simulink model "Controller_Disc2018"  (R2018b)
settings: Solver=ode8  StartTime=0.0  StopTime=100  FixedStep=1e-4  RelTol=1e-3
undefined symbols (not defined in the file or in its folder): DiscIntNeverNeededParam
libraries: simulink x2
settings Model: Creator=yarat  LastModifiedBy=uidr9910
settings SolverCC: AlgebraicLoopSolver=LineSearch
settings DataIOCC: ReturnWorkspaceOutputs=on

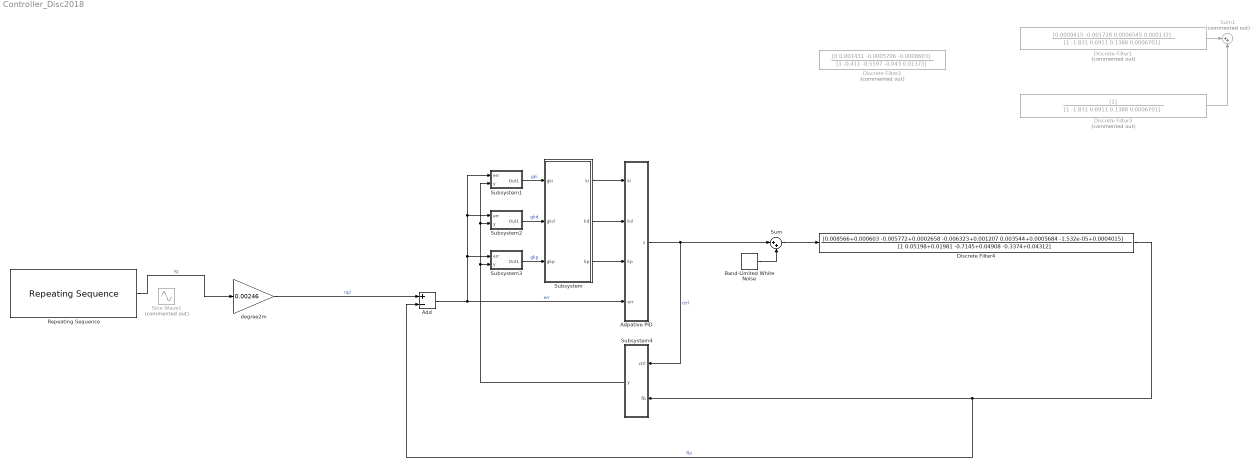
== system Controller_Disc2018 ==
  Add : Sum  Inputs=+-
  Adpative PID : Subsystem
  Band-Limited White Noise : simulink/Sources/Band-Limited White Noise  Cov=[0.00002]  Ts=0.1  seed=[23341]
  Discrete Filter1 : DiscreteFilter  Commented=on  Numerator=[0.0009415 -0.001728 0.0006545 0.000132]  Denominator=[1 -1.831 0.6911 0.1388 0.0006701]  FilterStructure=Direct form I  SampleTime=0.0001
  Discrete Filter2 : DiscreteFilter  Commented=on  Numerator=[0 0.001431 -0.0005706 -0.0008603]  Denominator=[1 -0.411 -0.5597 -0.043 0.01373]  FilterStructure=Direct form I  SampleTime=0.0001
  Discrete Filter3 : DiscreteFilter  Commented=on  Denominator=[1 -1.831 0.6911 0.1388 0.0006701]  FilterStructure=Direct form I  SampleTime=0.0001
  Discrete Filter4 : DiscreteFilter  Numerator=[0.008566+0.000603 -0.005772+0.0002658 -0.006323+0.001207 0.003544+0.0005684 -1.532e-05+0.0004015]  Denominator=[1 0.05198+0.01981 -0.7145+0.04908 -0.3374+0.04312]  FilterStructure=Direct form I  SampleTime=0.0001
  Repeating Sequence : simulink/Sources/Repeating Sequence  rep_seq_t=[0 3 3.01 6 6.01 9 9.01 12]*5  rep_seq_y=[1 1 0 0 -1 -1 0 0]*2
  Sine Wave1 : Sin  Commented=on  Amplitude=2  Frequency=0.5  SampleTime=0
  Subsystem : Subsystem
  Subsystem1 : Subsystem
  Subsystem2 : Subsystem
  Subsystem3 : Subsystem
  Subsystem4 : Subsystem
  Sum : Sum  Inputs=|++
  Sum1 : Sum  Commented=on  Inputs=|++
  degree2m : Gain  Gain=0.00246
  wires:
  degree2m/1 -> Add/1  "rq2"
  Add/1 -> Adpative PID/4(err), Subsystem1/1(err), Subsystem2/1(err), Subsystem3/1(err)  "err"
  Subsystem1/1(Out1) -> Subsystem/1(gki)  "gki"
  Subsystem2/1(Out1) -> Subsystem/2(gkd)  "gkd"
  Subsystem3/1(Out1) -> Subsystem/3(gkp)  "gkp"
  Subsystem/1(ki) -> Adpative PID/1(ki)
  Subsystem/2(kd) -> Adpative PID/2(kd)
  Subsystem/3(kp) -> Adpative PID/3(kp)
  Subsystem4/1(y) -> Subsystem3/2(y), Subsystem2/2(y), Subsystem1/2(y)
  Band-Limited White Noise/1 -> Sum/2
  Adpative PID/1(ctrl) -> Sum/1, Subsystem4/1(ctrl)  "ctrl"
  Sum/1 -> Discrete Filter4/1
  Discrete Filter4/1 -> Add/2, Subsystem4/2(fb)  "fbi"
  Repeating Sequence/1 -> degree2m/1  "rq"
  Discrete Filter1/1 -> Sum1/1
  Discrete Filter3/1 -> Sum1/2

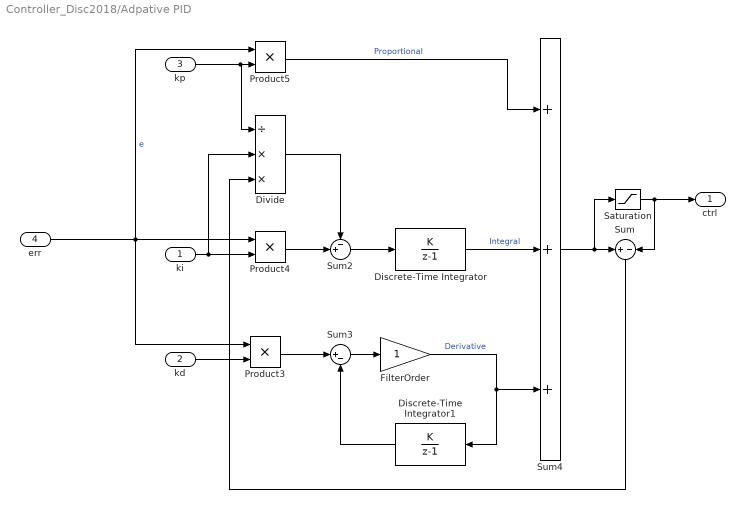
== system Controller_Disc2018/Adpative PID ==
  ki : Inport
  kd : Inport  Port=2
  kp : Inport  Port=3
  err : Inport  Port=4
  Discrete-Time Integrator : DiscreteIntegrator  IntegratorMethod=Accumulation: Forward Euler  gainval=0.001  SampleTime=-1  ICPrevOutput=DiscIntNeverNeededParam  ICPrevScaledInput=DiscIntNeverNeededParam
  Discrete-Time Integrator1 : DiscreteIntegrator  IntegratorMethod=Accumulation: Forward Euler  gainval=0.001  SampleTime=-1  ICPrevOutput=DiscIntNeverNeededParam  ICPrevScaledInput=DiscIntNeverNeededParam
  Divide : Product  Inputs=/**
  FilterOrder : Gain  SaturateOnIntegerOverflow=on  OutDataTypeStr=Inherit: Same as input  ParamDataTypeStr=Inherit: Same as input
  Product3 : Product
  Product4 : Product
  Product5 : Product
  Saturation : Saturate  UpperLimit=100  LowerLimit=-100
  Sum : Sum  Inputs=+|-
  Sum2 : Sum  Inputs=-+|
  Sum3 : Sum  Inputs=|+-
  Sum4 : Sum  Inputs=+++  InputSameDT=on  SaturateOnIntegerOverflow=on  OutDataTypeStr=Inherit: Same as first input
  ctrl : Outport
  wires:
  Discrete-Time Integrator/1 -> Sum4/2  "Integral"
  Discrete-Time Integrator1/1 -> Sum3/2
  Sum/1 -> Divide/3
  Sum2/1 -> Discrete-Time Integrator/1
  Product3/1 -> Sum3/1
  Sum3/1 -> FilterOrder/1
  Product4/1 -> Sum2/2
  FilterOrder/1 -> Sum4/3, Discrete-Time Integrator1/1  "Derivative"
  Product5/1 -> Sum4/1  "Proportional"
  Saturation/1 -> ctrl/1, Sum/2
  err/1 -> Product4/1, Product3/1, Product5/1  "e"
  Sum4/1 -> Saturation/1, Sum/1
  kp/1 -> Divide/1, Product5/2
  ki/1 -> Product4/2, Divide/2
  kd/1 -> Product3/2
  Divide/1 -> Sum2/1

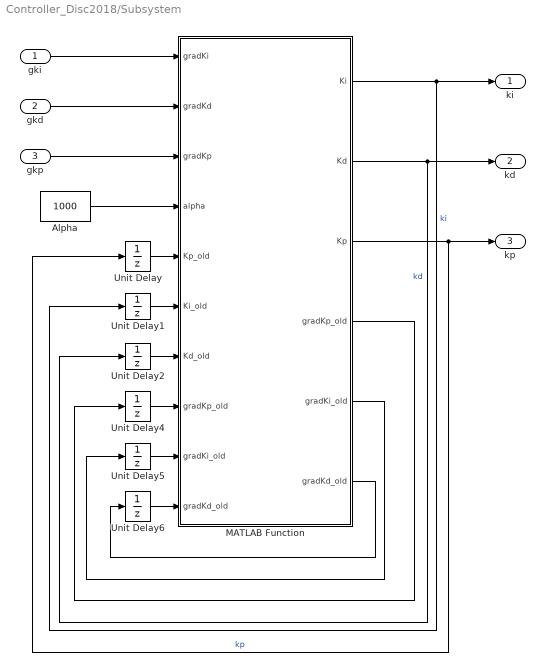
== system Controller_Disc2018/Subsystem ==
  gki : Inport
  gkd : Inport  Port=2
  gkp : Inport  Port=3
  Alpha : Constant  Value=1000
  MATLAB Function : MATLAB Function  TreatAsAtomicUnit=on
  Unit Delay : UnitDelay  InitialCondition=800  SampleTime=1e-3  HasFrameUpgradeWarning=on
  Unit Delay1 : UnitDelay  InitialCondition=300  SampleTime=1e-3  HasFrameUpgradeWarning=on
  Unit Delay2 : UnitDelay  InitialCondition=4  SampleTime=1e-3  HasFrameUpgradeWarning=on
  Unit Delay4 : UnitDelay  SampleTime=1e-3  HasFrameUpgradeWarning=on
  Unit Delay5 : UnitDelay  SampleTime=1e-3  HasFrameUpgradeWarning=on
  Unit Delay6 : UnitDelay  SampleTime=1e-3  HasFrameUpgradeWarning=on
  ki : Outport
  kd : Outport  Port=2
  kp : Outport  Port=3
  wires:
  Unit Delay4/1 -> MATLAB Function/8("gradKp_old ")
  MATLAB Function/2(Kd) -> kd/1, Unit Delay2/1  "kd"
  MATLAB Function/6(gradKd_old) -> Unit Delay6/1
  Unit Delay1/1 -> MATLAB Function/6(Ki_old)
  MATLAB Function/4(gradKp_old) -> Unit Delay4/1
  Alpha/1 -> MATLAB Function/4(alpha)
  MATLAB Function/5(gradKi_old) -> Unit Delay5/1
  MATLAB Function/3(Kp) -> kp/1, Unit Delay/1  "kp"
  Unit Delay6/1 -> MATLAB Function/10("gradKd_old ")
  Unit Delay/1 -> MATLAB Function/5(Kp_old)
  MATLAB Function/1(Ki) -> ki/1, Unit Delay1/1  "ki"
  Unit Delay5/1 -> MATLAB Function/9("gradKi_old ")
  Unit Delay2/1 -> MATLAB Function/7(Kd_old)
  gki/1 -> MATLAB Function/1(gradKi)
  gkd/1 -> MATLAB Function/2(gradKd)
  gkp/1 -> MATLAB Function/3(gradKp)

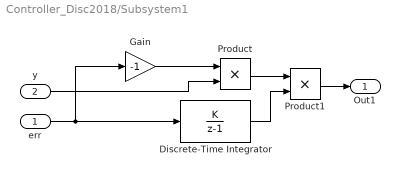
== system Controller_Disc2018/Subsystem1 ==
  err : Inport
  y : Inport  Port=2
  Discrete-Time Integrator : DiscreteIntegrator  IntegratorMethod=Accumulation: Forward Euler  gainval=0.0001  SampleTime=-1  ICPrevOutput=DiscIntNeverNeededParam  ICPrevScaledInput=DiscIntNeverNeededParam
  Gain : Gain  Gain=-1
  Product : Product
  Product1 : Product
  Out1 : Outport
  wires:
  Discrete-Time Integrator/1 -> Product1/2
  Gain/1 -> Product/1
  Product1/1 -> Out1/1
  Product/1 -> Product1/1
  y/1 -> Product/2
  err/1 -> Discrete-Time Integrator/1, Gain/1

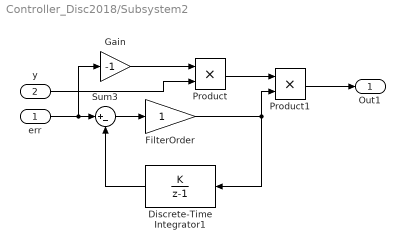
== system Controller_Disc2018/Subsystem2 ==
  err : Inport
  y : Inport  Port=2
  Discrete-Time Integrator1 : DiscreteIntegrator  IntegratorMethod=Accumulation: Forward Euler  gainval=0.0001  SampleTime=-1  ICPrevOutput=DiscIntNeverNeededParam  ICPrevScaledInput=DiscIntNeverNeededParam
  FilterOrder : Gain  SaturateOnIntegerOverflow=on  OutDataTypeStr=Inherit: Same as input  ParamDataTypeStr=Inherit: Same as input
  Gain : Gain  Gain=-1
  Product : Product
  Product1 : Product
  Sum3 : Sum  Inputs=|+-
  Out1 : Outport
  wires:
  y/1 -> Product/2
  Product/1 -> Product1/1
  Product1/1 -> Out1/1
  Gain/1 -> Product/1
  err/1 -> Sum3/1, Gain/1
  Sum3/1 -> FilterOrder/1
  Discrete-Time Integrator1/1 -> Sum3/2
  FilterOrder/1 -> Discrete-Time Integrator1/1, Product1/2

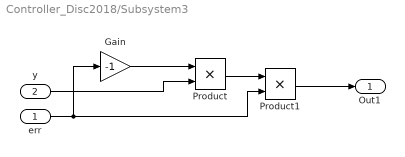
== system Controller_Disc2018/Subsystem3 ==
  err : Inport
  y : Inport  Port=2
  Gain : Gain  Gain=-1
  Product : Product
  Product1 : Product
  Out1 : Outport
  wires:
  Gain/1 -> Product/1
  Product1/1 -> Out1/1
  Product/1 -> Product1/1
  y/1 -> Product/2
  err/1 -> Gain/1, Product1/2

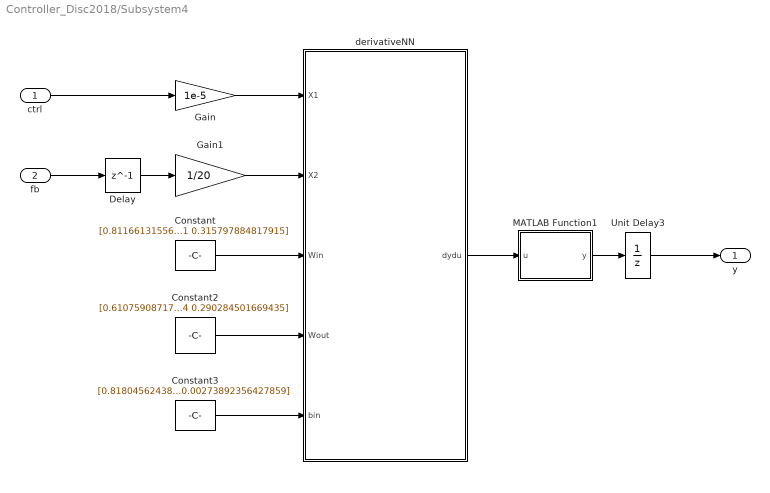
== system Controller_Disc2018/Subsystem4 ==
  ctrl : Inport
  fb : Inport  Port=2
  Constant : Constant  Value=|
      | [0.811661315567532	0.523339604043497
      | 0.781547366351639	0.164018692936968
      | 0.146098503423341	0.879428705628321
      | 0.266102211582170	0.304501614309624
      | 0.397284814093776	0.765244619952808
      | 0.516628753495178	0.186405621841320
      | 0.0862525926601981	0.717804970916536
      | 0.103414091455425	0.420647287190983
      | 0.506698658207659	0.609237422549281
      | 0.269175608561842	0.124471251020265
      | 0.0151134208657587	0.418749009267761
      | 0.873047701593747	0.980270684978551
      | 0.0624305176835148	0.302769416201919
      | 0.0444243510475763	0.430246616185495
      | 0.956127765123271	0.142311041042483
      | 0.549202286331316	0.311122631590002
      | 0.713499976100381	0.159301438083396
      | 0.328775895527325	0.385292704689736
      | 0.649001722373211	0.236663924286235
      | 0.0654762342586071	0.315797884817915]
  Constant2 : Constant  Value="[0.610759087177597\t0.366179666335005\t-0.0584030572951834\t0.209075859992505\t0.584389586358981\t0.349871470561781\t-0.204405272265807\t-0.116182445469499\t0.0642557952818070\t-0.132902026263845\t0.805831183296775\t-0.399691016290584\t0.259161704540015\t0.179474388613012\t-0.0314937390524749\t0.704808744971737\t0.263155510958995\t0.213381634610559\t0.587918070221544\t0.290284501669435]"
  Constant3 : Constant  Value=|
      | [0.818045624381218
      | 0.102878023447675
      | 0.737296135799067
      | 0.382188425410472
      | 0.977505309905872
      | 0.149360203196300
      | 0.641439600546557
      | 0.443497484934195
      | 0.680421925309724
      | 0.859879825832941
      | -0.318689482669828
      | 0.255207188653107
      | 0.313389787503390
      | 0.721063295306122
      | 0.439116073494923
      | -0.219038629148731
      | 0.491813043211072
      | -0.0750940652226708
      | -0.120979967962816
      | 0.00273892356427859]
  Delay : Delay  DelayLength=1  SampleTime=1e-3
  Gain : Gain  Gain=1e-5
  Gain1 : Gain  Gain=1/20
  MATLAB Function1 : MATLAB Function  TreatAsAtomicUnit=on
  Unit Delay3 : UnitDelay  SampleTime=1e-3  HasFrameUpgradeWarning=on
  derivativeNN : MATLAB Function  TreatAsAtomicUnit=on
  y : Outport
  wires:
  Gain/1 -> derivativeNN/1(X1)
  derivativeNN/1(dydu) -> MATLAB Function1/1(u)
  Constant2/1 -> derivativeNN/4(Wout)
  Constant/1 -> derivativeNN/3(Win)
  Constant3/1 -> derivativeNN/5(bin)
  Delay/1 -> Gain1/1
  Gain1/1 -> derivativeNN/2(X2)
  MATLAB Function1/1(y) -> Unit Delay3/1
  ctrl/1 -> Gain/1
  Unit Delay3/1 -> y/1
  fb/1 -> Delay/1

== matlab function Controller_Disc2018/Subsystem4/derivativeNN ==
  data: X1 input size=[1,1]; X2 input size=[1,1]; dydu output size=[1,1]; Win input size=[20,2]; Wout input size=[1,20]; bin input size=[20,1]

function dydu  = ffnetforcast(X1,X2, Win, Wout, bin)
X = [X1;X2];
netin = Win*X + bin;
dydu_pre = Win'*(Wout'.*hprime(netin));
dydu = dydu_pre(1,1);
function y = hprime(x)
    y = (1-tanh(x).^2);
end
end

== matlab function Controller_Disc2018/Subsystem/MATLAB Function ==
  data: gradKi input; Ki output; gradKd input; gradKp input; Kd output; Kp output; alpha input; Kp_old input; Ki_old input; Kd_old input; gradKp_old input; gradKi_old input; gradKd_old input; gradKp_old output; gradKi_old output; gradKd_old output
function [Ki,Kd,Kp,gradKp_old,gradKi_old,gradKd_old] = fcn(gradKi,gradKd,gradKp, alpha, Kp_old, Ki_old, Kd_old,gradKp_old,gradKi_old,gradKd_old)



% v = beta*(oldGrad) + (1-beta)*grad;
% oldGrad = v;
% param = param - alpha*v;
beta = 0.8;
Vkp = beta*gradKp_old + (1-beta)*gradKp;
Vki = beta*gradKi_old + (1-beta)*gradKi;
Vkd = beta*gradKd_old + (1-beta)*gradKd;

Kp = Kp_old - alpha*Vkp;
Ki = Ki_old - alpha*Vki;
Kd = Kd_old - alpha*Vkd;

gradKp_old = Vkp;
gradKi_old = Vki;
gradKd_old = Vkd;


end

== matlab function Controller_Disc2018/Subsystem4/MATLAB Function1 ==
  data: u input; y output
function y = fcn(u)
if u == 0
    y = 0.0001;
else
y = u;
end
